simulink model "rad_ut"  (Simulink 8.1)
settings: Solver=ode1  StartTime=0.0  StopTime=Inf  FixedStep=0.001  RelTol=1e-3
PostLoadFcn:
  | , if any(exist('dsrtsu_mdlpostloadfcn', 'file') == [2, 3, 6]), try dsrtsu_mdlpostloadfcn('Execute', bdroot); catch fprintf('Error in PostLoadFcn (dsrtsu_mdlpostloadfcn) for model "%s":\n %s\n', bdroot, lasterr); end, end,
libraries: siltestlib x7, rad x1
settings Model: DSRTSU_INTERNAL_RTI_VER=450  DSRTSU_INTERNAL_RTI_TYPE=rti1401  RTICANMMDATA=struct('GeneralSetupData',struct('modelroot','D:\PROJECTS\HAITEC\IDIADA_SVN\TEAM\TEscamilla\Project1\AdasDragon\software\sw_development\arch\app\per\rad','generalsettings',struct('filesettings',struct('destfolder',struct('Name','RTICANMM_FILES','Check',1),'buildfolder',struct('Name','.','Check',1),'AbsDestfolder',struct('Name','D:\PROJECTS\HAITEC\IDIADA_SVN\TEAM\TEscamilla\Project1\AdasDragon\software\sw_development\arch\app\per\rad\RTICANMM_FILES'),'AbsBuildfolder',struct('Name','D:\PROJECTS\HAITEC\IDIADA_SVN\TEAM\TEscamilla\Project1\AdasDragon\software\sw_development\arch\app\per\rad'))),'options',struct('addpaths',1,'rmpaths',1,'addtrcexclusion',logical(1),'cannavigator',struct('checkmonitoring',0),'show_usrtrc',0,'use_usrtrc',0),'advanced',struct('options',[1 1 1 1 1 1 1 1 1 1 1 1 1 1 1 1 1 1 1 1 1 1 1 1 1 1 1 1 1 1 1 1 1 1 1 1 1 1 1 1 1 1 1 1 1 1 1 1 1 1 1 1 1 1 1 1 1 1 1 1 1 1 1 1 1 1 1 1 1 1 1 1 1 1 1 1 1 1 1 1 1 1 1 1 1 1 1 1 1 1 1 1 1 1 1 1 1 1 1 1]),'MPSetup',{{}},'modelname','rad_ut','block','rad_ut'))  DSRTSU_INTERNAL_RTIFPGA=40  Creator=tescamilla  LastModifiedBy=tescamilla  BufferReuse=off
settings DataIOCC: SignalLoggingSaveFormat=Dataset
settings OptimizationCC: BlockReduction=off  OptimizeBlockIOStorage=off  BufferReuse=off  ExpressionFolding=off  ExpressionDepthLimit=128  LocalBlockOutputs=off
settings DebuggingCC: FcnCallInpInsideContextMsg=EnableAllAsError
settings HardwareCC: ProdIntDivRoundTo=Zero  ProdEndianess=BigEndian  ProdHWDeviceType=Generic->Custom  TargetIntDivRoundTo=Zero  TargetEndianess=BigEndian  TargetHWDeviceType=Generic->Custom
settings RTWCC: SystemTargetFile=rti1401.tlc  MakeCommand=make_rti  TemplateMakefile=rti1401.tmf  Description=dSPACE DS1401 Hardware Platform  ProcessScript=rti1401_make_rtw_hook
settings STFCustomTargetCC: CodeReplacementLibrary=ANSI_C  ParMdlRefBuildCompliant=on  GeneratePreprocessorConditionals=Disable all  MatFileLogging=on  SystemTargetFile=rti1401.tlc
settings GRTTargetCC: CompOptLevelCompliant=off  ConcurrentExecutionCompliant=off  ExtModeMexFile=noextcomm
settings CustomProperty: DataType=RTWOptions_EnumType_C__Program Files (x86)_dSPACE RCPHIL 2014-B_MATLAB_RTI_RTI1401_TLC_rti1401_1InitialSimState  Value=RUN
settings EnumStrPairs: String=RUN

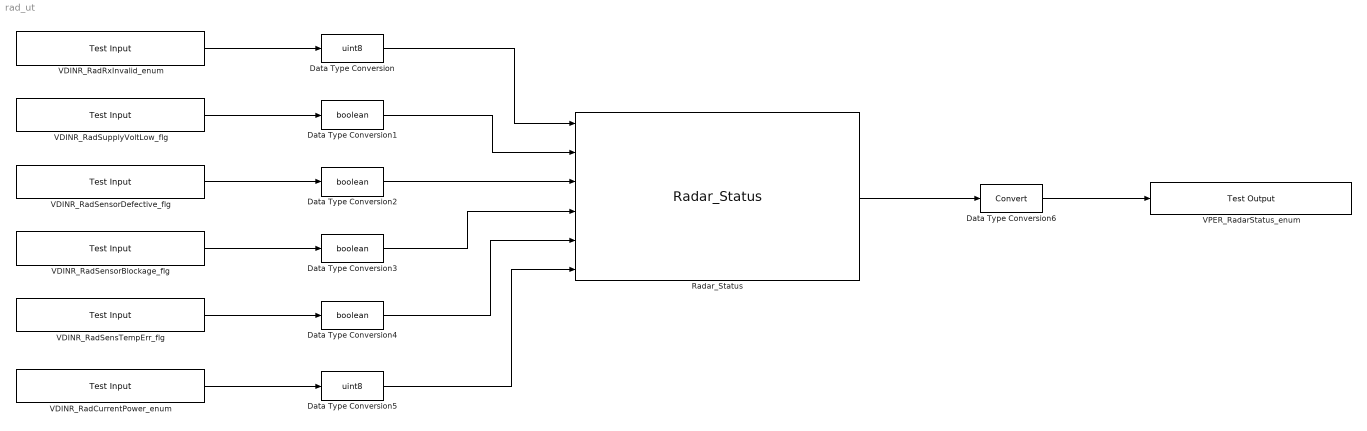
== system rad_ut ==
  Data Type Conversion : DataTypeConversion  OutDataTypeStr=uint8
  Data Type Conversion{1..4} (4 alike) : DataTypeConversion  OutDataTypeStr=boolean
  Data Type Conversion5 : DataTypeConversion  OutDataTypeStr=uint8
  Data Type Conversion6 : DataTypeConversion
  Radar_Status : rad/Radar_Status
  VDINR_RadCurrentPower_enum : siltestlib/Test Input  varname=VDINR_RadCurrentPower_enum  sampletime=-1
  VDINR_RadRxInvalid_enum : siltestlib/Test Input  varname=VDINR_RadRxInvalid_enum  sampletime=-1
  VDINR_RadSensTempErr_flg : siltestlib/Test Input  varname=VDINR_RadSensTempErr_flg  sampletime=-1
  VDINR_RadSensorBlockage_flg : siltestlib/Test Input  varname=VDINR_RadSensorBlockage_flg  sampletime=-1
  VDINR_RadSensorDefective_flg : siltestlib/Test Input  varname=VDINR_RadSensorDefective_flg  sampletime=-1
  VDINR_RadSupplyVoltLow_flg : siltestlib/Test Input  varname=VDINR_RadSupplyVoltLow_flg  sampletime=-1
  VPER_RadarStatus_enum : siltestlib/Test Output  varname=VPER_RadarStatus_enum  sampletime=-1
  wires:
  VDINR_RadRxInvalid_enum/1 -> Data Type Conversion/1
  VDINR_RadSupplyVoltLow_flg/1 -> Data Type Conversion1/1
  VDINR_RadSensorDefective_flg/1 -> Data Type Conversion2/1
  VDINR_RadSensorBlockage_flg/1 -> Data Type Conversion3/1
  VDINR_RadSensTempErr_flg/1 -> Data Type Conversion4/1
  VDINR_RadCurrentPower_enum/1 -> Data Type Conversion5/1
  Radar_Status/1 -> Data Type Conversion6/1
  Data Type Conversion/1 -> Radar_Status/1
  Data Type Conversion1/1 -> Radar_Status/2
  Data Type Conversion2/1 -> Radar_Status/3
  Data Type Conversion3/1 -> Radar_Status/4
  Data Type Conversion4/1 -> Radar_Status/5
  Data Type Conversion5/1 -> Radar_Status/6
  Data Type Conversion6/1 -> VPER_RadarStatus_enum/1
